simulink model "StabObserFlou"  (R2017a)
settings: Solver=VariableStepAuto  StartTime=0.0  StopTime=5  RelTol=1e-3
values from neighbouring files (symbols this model uses):
  B = 1    [Animation.m]    (also in Model.m = [0 ; 1/tau])
  C = [tr+(f*n1) 0]    [Model.m]
  K = NaN    [FctPP.m]    (also in Gainfind.m; GainfindV2.m; GainfindVTD.m = struct('matrix',{zeros(m,n)}); Mainscript.m = cat(3,K(1:r).matrix))
  L = 4    [Animation.m]    (also in Mainscript.m = cat(3,L(1:r).matrix); Observateurflou.m = NaN)
  Parametres = [ax, bx, Rap, alpha, tau]    [Model.m]
  Parametres2 = [tr, f]    [Model.m]
undefined symbols (not defined in the file or in its folder): A
settings Model: Creator=MONCEF  LastModifiedBy=MONCEF

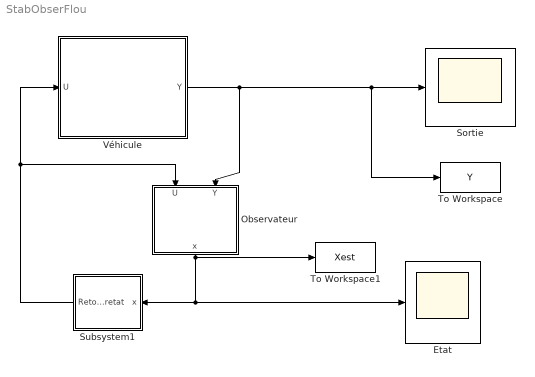
== system StabObserFlou ==
  Etat : Scope
  Observateur : Subsystem
  Sortie : Scope
  Subsystem1 : Subsystem
  To Workspace : ToWorkspace  VariableName=Y  SaveFormat=Structure With Time  SampleTime=0.001
  To Workspace1 : ToWorkspace  VariableName=Xest  SaveFormat=Structure With Time  SampleTime=0.001
  Véhicule : Subsystem
      mask Display: image(fullfile(pwd,'Images','VehiculeSuiveur.jpg'));
  wires:
  Véhicule/1(Y) -> To Workspace/1, Sortie/1, Observateur/2(Y)
  Observateur/1(x) -> Etat/1, Subsystem1/1(x), To Workspace1/1
  Subsystem1/1(Retouretat) -> Véhicule/1(U), Observateur/1(U)

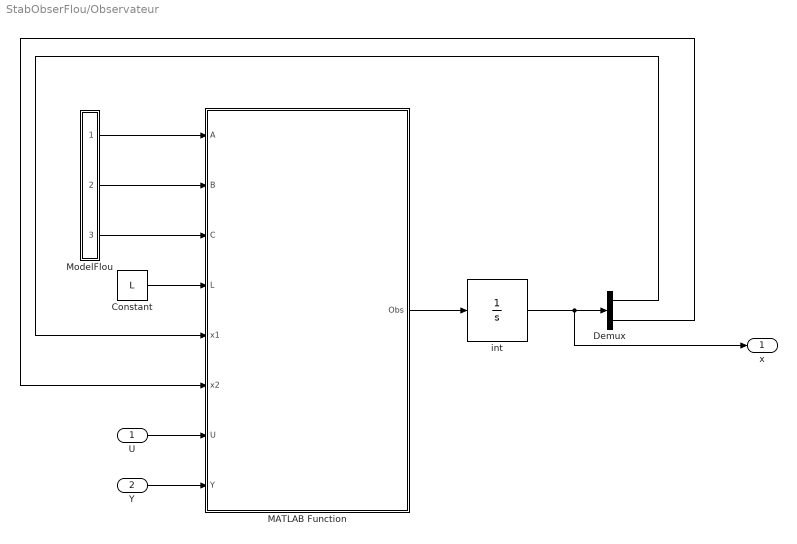
== system StabObserFlou/Observateur ==
  U : Inport
  Y : Inport  Port=2
  Constant : Constant  Value=L
  Demux : Demux  Outputs=2
  MATLAB Function : MATLAB Function  TreatAsAtomicUnit=on
  ModelFlou : Subsystem
  int : Integrator  InitialCondition=[5 3]
      mask Display: image(fullfile(pwd,'Images','Integrateur.png'));
  x : Outport
  wires:
  MATLAB Function/1(Obs) -> int/1
  Demux/2 -> MATLAB Function/6(x2)
  Demux/1 -> MATLAB Function/5(x1)
  int/1 -> Demux/1, x/1
  U/1 -> MATLAB Function/7(U)
  Y/1 -> MATLAB Function/8(Y)
  Constant/1 -> MATLAB Function/4(L)
  ModelFlou/1(A) -> MATLAB Function/1(A)
  ModelFlou/2(B) -> MATLAB Function/2(B)
  ModelFlou/3(C) -> MATLAB Function/3(C)

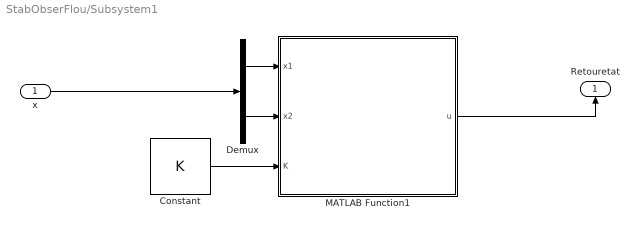
== system StabObserFlou/Subsystem1 ==
  x : Inport
  Constant : Constant  Value=K
  Demux : Demux  Outputs=2
  MATLAB Function1 : MATLAB Function  TreatAsAtomicUnit=on
  Retouretat : Outport
  wires:
  Constant/1 -> MATLAB Function1/3(K)
  x/1 -> Demux/1
  Demux/2 -> MATLAB Function1/2(x2)
  Demux/1 -> MATLAB Function1/1(x1)
  MATLAB Function1/1(u) -> Retouretat/1

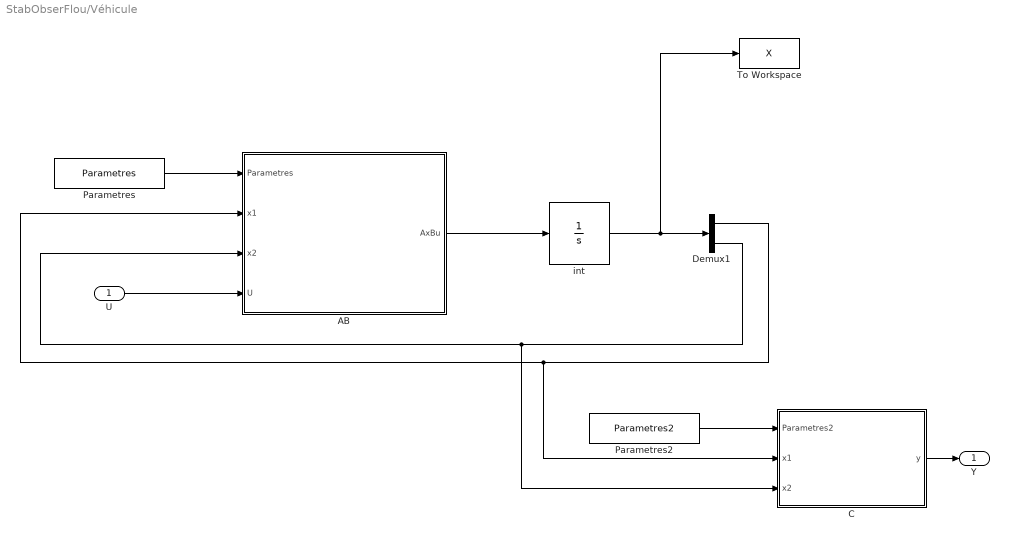
== system StabObserFlou/Véhicule ==
  U : Inport
  AB : MATLAB Function  TreatAsAtomicUnit=on
  C : MATLAB Function  TreatAsAtomicUnit=on
  Demux1 : Demux  Outputs=2
  Parametres : Constant  Value=Parametres
  Parametres2 : Constant  Value=Parametres2
  To Workspace : ToWorkspace  VariableName=X  SaveFormat=Structure With Time  SampleTime=0.001
  int : Integrator  InitialCondition=[1 1]
      mask Display: image(fullfile(pwd,'Images','Integrateur.png'));
  Y : Outport
  wires:
  C/1(y) -> Y/1
  Parametres/1 -> AB/1(Parametres)
  Parametres2/1 -> C/1(Parametres2)
  U/1 -> AB/4(U)
  AB/1(AxBu) -> int/1
  Demux1/2 -> C/3(x2), AB/3(x2)
  Demux1/1 -> C/2(x1), AB/2(x1)
  int/1 -> To Workspace/1, Demux1/1

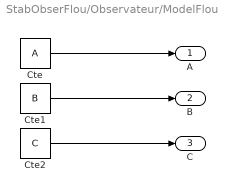
== system StabObserFlou/Observateur/ModelFlou ==
  Cte : Constant  Value=A
  Cte1 : Constant  Value=B
  Cte2 : Constant  Value=C
  A : Outport
  B : Outport  Port=2
  C : Outport  Port=3
  wires:
  Cte1/1 -> B/1
  Cte2/1 -> C/1
  Cte/1 -> A/1

== matlab function StabObserFlou/Véhicule/AB ==
  data: Parametres input; x1 input; AxBu output; x2 input; U input
function AxBu = fcn(Parametres,x1,x2,U)

ax = Parametres(1);
bx = Parametres(2);
Rap = Parametres(3);
alpha = Parametres(4);
tau = Parametres(5);

%define the systeme matrix
A =[-(ax+bx*x1)/alpha Rap/alpha; 0 -1/tau];
B =[0 ; 1/tau];



AxBu = A*[x1;x2]+B*U;

== matlab function StabObserFlou/Observateur/MATLAB Function ==
  data: A input; B input; C input; L input; x1 input; Obs output; x2 input; U input; Y input
function Obs = fcn(A,B,C,L,x1,x2,U,Y)
x=[x1; x2];
T1 = (x1-2)/(25-2);
T2 = (25-x1)/(25-2);
%%
L1 = L(:,:,1);
L2 = L(:,:,2);

%%
%define the systeme matrix
A1 = A(:,:,1);
B1 = B(:,:,1);
C1 = C(:,:,1);

A2 = A(:,:,2);
B2 = B(:,:,2);
C2 = C(:,:,2);

%%
yo = (T1*C1+T2*C2)*x;

%%

A1xB1uL1e = A1*x+B1*U+L1*(Y-yo);
A2xB2uL2e = A2*x+B2*U+L2*(Y-yo);

Obs = T1*A1xB1uL1e +T2*A2xB2uL2e;

== matlab function StabObserFlou/Subsystem1/MATLAB Function1 ==
  data: x1 input; x2 input; u output; K input
function u = fcn(x1,x2,K)

x=[x1;x2];

K1=K(:,:,1);
K2=K(:,:,2);



T1 =(x1-0)/(100);
T2 =(100-x1)/(100);

u =-(T1*K1+T2*K2)*x;

== matlab function StabObserFlou/Véhicule/C ==
  data: Parametres2 input; x1 input; y output; x2 input
function y = fcn(Parametres2,x1,x2)
tr = Parametres2(1);
f = Parametres2(2);

C = [tr+f*x1 0];
y =C*[x1;x2];
